simulink model "SPARCS_MIL"  (R2024a)
settings: Solver=VariableStepAuto  StartTime=0.0  StopTime=10.0  RelTol=1e-3
undefined symbols (not defined in the file or in its folder): attitude, epoch, IAU, juliandate, km, m, om0_x, om0_y, om0_z, s, satellite, simulator, WMM2020
libraries: simulink_extras x16, sharedtransform x14, SepehrMILLib x10, aerolibconvert2 x9, matrix_library x3, simulink x3, aerolibutil x3, vrlib x2, aerolibgravity2 x2, aerolibtransform2 x2
(part 1 of 2)
settings Model: Creator=dani  LastModifiedBy=dani

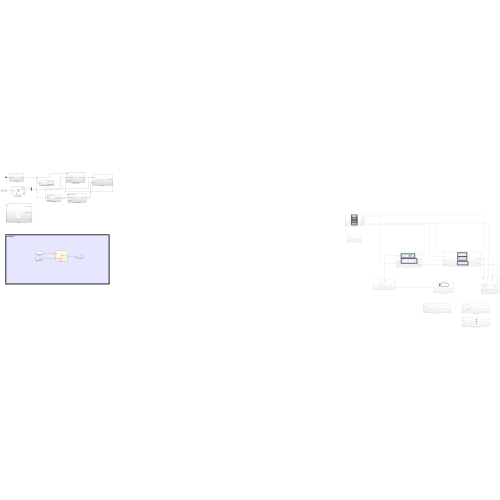
[thumbnail: Simulink's stored preview of the top-level diagram]
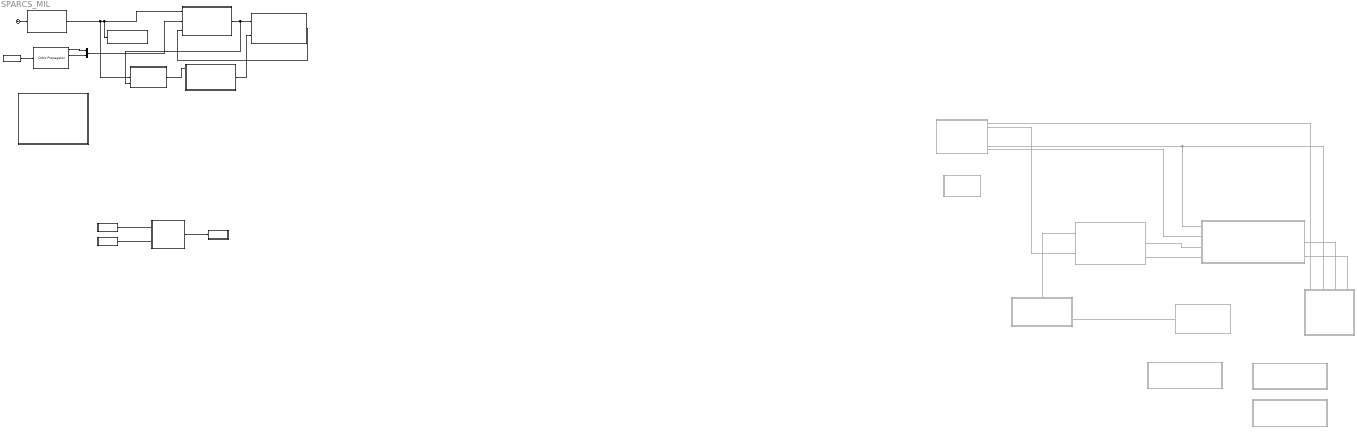
== system SPARCS_MIL ==
  note: Software
  Actuators : Subsystem  Commented=on
      settings: PortSchema="{\"entries\":[{\"content\":{\"sides\":[{\"content\":{},\"type\":\"ConnectorPlacement.EquallySpacedRectSide\",\"uuid\":\"57b5be20-0305-4655-b70d-f6d88ddf7cc3\"},{\"content\":{\"connectorIds\":[\"In1\",\"In2\"],\"side\":\"RIGHT\"},\"type\":\"ConnectorPlacement.EquallySpacedRectSide\",\"uuid\":\"30fbf78c-d5a5-42a2-90f1-8bab57c6ab77\"},{\"content\":{\"connectorIds\":[\"Out1\"],\"side\":\"TOP\"},\"type\":\"ConnectorPlacement.EquallySpacedRectSide\",\"uuid\":\"5a8d2e79-d609-4b0c-a176-c302cc1b65d1\"}]},\"type\":\"ConnectorPlacement.EquallySpacedConnector\",\"uuid\":\"3b08abd5-9373-451e-94da-caa467f9d6bd\"}],\"packageUris\":[\"http://schema.mathworks.com/mf0/Connector/R2020b\"],\"version\":\"1.0\"}"
  Attitude Control Algorithms : Subsystem  Commented=on
      settings: PortSchema="{\"entries\":[{\"content\":{\"sides\":[{\"content\":{\"connectorIds\":[\"Out1\"]},\"type\":\"ConnectorPlacement.EquallySpacedRectSide\",\"uuid\":\"41f8dcfc-afb1-4613-bda0-8bd0e5f6db23\"},{\"content\":{\"side\":\"RIGHT\"},\"type\":\"ConnectorPlacement.EquallySpacedRectSide\",\"uuid\":\"1cc831b3-3219-4888-a8b3-e3dddebb1701\"},{\"content\":{\"side\":\"TOP\"},\"type\":\"ConnectorPlacement.EquallySpacedRectSide\",\"uuid\":\"ddd3243b-04bb-419c-9fbc-88ec0dbe35ac\"}]},\"type\":\"ConnectorPlacement.EquallySpacedConnector\",\"uuid\":\"03796cc2-c9a7-47b9-b2cd-c3bab7a65dae\"}],\"packageUris\":[\"http://schema.mathworks.com/mf0/Connector/R2020b\"],\"version\":\"1.0\"}"
  Attitude Determination and Estimation Algorithms : Subsystem  Commented=on
      settings: PortSchema="{\"entries\":[{\"content\":{\"sides\":[{\"content\":{\"connectorIds\":[\"Out1\",\"Out2\",\"Out3\"]},\"type\":\"ConnectorPlacement.EquallySpacedRectSide\",\"uuid\":\"7b05d57f-a0cf-4401-a574-34b1755f21cb\"},{\"content\":{\"side\":\"RIGHT\"},\"type\":\"ConnectorPlacement.EquallySpacedRectSide\",\"uuid\":\"0f587f50-2c0a-47b1-bbff-e10884228d7f\"},{\"content\":{\"connectorIds\":[\"In1\",\"In2\",\"In3\",\"In4\"],\"side\":\"TOP\"},\"type\":\"ConnectorPlacement.EquallySpacedRectSide\",\"uuid\":\"7d75d2d9-c6c8-4539-b1b4-022bd2bc80cb\"},{\"content\":{\"side\":\"BOTTOM\"},\"type\":\"ConnectorPlacement.EquallySpacedRectSide\",\"uuid\":\"9e386f38-6887-4261-b78f-0a16f9b94efd\"}]},\"type\":\"ConnectorPlacement.EquallySpacedConnector\",\"uuid\":\"071a0923-cd7c-4dcb-a7b9-f4842b9df63f\"}],\"packageUris\":[\"http://schema.mathworks.com/mf0/Connector/R2020b\"],\"version\":\"1.0\"}"
  Attitude Dynamic : Subsystem
  Bus Creator : BusCreator  Inputs=2
  Calendar : Subsystem
  Clock : Clock
  Constant : Constant  Value=[0; 0; 0]
  Environment : Subsystem  Commented=on
  GNSS Receiver Model : Subsystem  Commented=on
  Gyroscope Model : Subsystem  Commented=on
  IGRF [ECEF] : Subsystem
  Kinematics and Dynamics : Subsystem  Commented=on
  Magnetometer Model : Subsystem  Commented=on
  Magnetorquers Model : Subsystem
  OBC : Stateflow chart  TreatAsAtomicUnit=on
  Orbit Propagator Numerical (high precision) : OrbitPropagator  propagator=Numerical (high precision)  accelIn=on  startDate=juliandate(epoch.Year, epoch.Month, epoch.Day, epoch.Hour, epoch.Minute, epoch.Second)  orbitType=Circular inclined  semiMajorAxis=6921000  inclination=55  raan=0  inertialPosition=[3649700.0 3308200.0 -4676600.0]  inertialVelocity=[-2750.8 6666.4 2573.4]  fixedPosition=[-4142689.0 -2676864.7 -4669861.6]  fixedVelocity=[1452.7 -6720.7 2568.1]  customR=3396200  customMu=4.305e13  customJ2=1.0826269e-03  customOmega=4.06125949e-3  outputTransform=on
  Planetary Ephemeris Calculator : Subsystem
  Reference Frames Transformations Manager : Subsystem
  Sensors : Subsystem
  Sensors1 : Subsystem  Commented=on
  Subsystem3 : Subsystem  Commented=on
  sensors sim : Subsystem
  telecommand receiver : Subsystem
  telemetry transponder : Subsystem
  wires:
  Environment/2(T_D(Body)) -> Kinematics and Dynamics/2(T_D(body))
  Kinematics and Dynamics/3(Omega(Body)[rad/s]) -> Sensors1/4(Omega(Body)[rad/s])
  Kinematics and Dynamics/2(q(ECI-Body)) -> Sensors1/3(q(ECI-Body))
  Environment/7(SunPos(ECI)) -> Attitude Determination and Estimation Algorithms/2(SunPos(ECI)), Sensors1/1(SunPos(ECI))
  Sensors1/2(B_meas(Body)[T]) -> Attitude Determination and Estimation Algorithms/3(B_Meas(Body))
  Sensors1/3(SunPos_Meas(Body)) -> Attitude Determination and Estimation Algorithms/4(SunPos_Meas(Body))
  Environment/8(Eclipse) -> Sensors1/2(Eclipse)
  Actuators/1(T_C(Body)) -> Kinematics and Dynamics/1(T_C(body))
  Environment/1(B(ECI)) -> Attitude Determination and Estimation Algorithms/1(B(ECI)[T])
  Attitude Control Algorithms/1(m) -> Actuators/2(m)
  Clock/1 -> Calendar/1(Since Epoch (sec))
  Calendar/1(Calendar) -> IGRF [ECEF]/2(Calendar), Planetary Ephemeris Calculator/1(Calendar), Reference Frames Transformations Manager/1(Calendar)
  Constant/1 -> Orbit Propagator Numerical (high precision)/1
  Orbit Propagator Numerical (high precision)/1 -> Bus Creator/1  "X"
  Orbit Propagator Numerical (high precision)/2 -> Bus Creator/2  "Y"
  Bus Creator/1 -> Reference Frames Transformations Manager/2(Ephemerides [ICRF])
  Reference Frames Transformations Manager/1(Transformers) -> IGRF [ECEF]/3(Transformers), Attitude Dynamic/1(Transformers)
  Attitude Dynamic/1(Satellite Attitude) -> Reference Frames Transformations Manager/3(Satellite Attitude)
  IGRF [ECEF]/1(Magnetic Field (T)) -> Magnetorquers Model/1(Magnetic Field [Body] (T))  "Magnetic Field (T)"
  Magnetorquers Model/1(Magnetorquers) -> Attitude Dynamic/2(Actuators)  "MTQs"
  sensors sim/1(Out1) -> OBC/1(sensors)
  telecommand receiver/1(telecommand) -> OBC/2(telecommand)
  OBC/1(telemetry) -> telemetry transponder/1(In1)

== system SPARCS_MIL/Actuators ==
  B(Body) : Inport
  m : Inport  Port=2
  A1 : Constant
  A2 : Constant
  Ax : Constant
  Cross Product : matrix_library/Cross Product
  Cross Product1 : matrix_library/Cross Product
  Cross Product2 : matrix_library/Cross Product
  Demux : Demux  Outputs=3
  Divide : Product  Inputs=*/
  Divide1 : Product  Inputs=*/
  Divide2 : Product  Inputs=*/
  Mux : Mux  Inputs=3
  N*A : Product
  N*A1 : Product
  N*A2 : Product
  N2 : Constant
  Nx : Constant
  Ny : Constant
  PWM : simulink/Discontinuities/PWM  DisableCoverage=on  Period=1  InitialDelay=0  DisallowZeroDutyCycle=off  RunAtFixedTimeIntervals=off  SampleTime=0.1
  PWM1 : simulink/Discontinuities/PWM  DisableCoverage=on  Period=1  InitialDelay=0  DisallowZeroDutyCycle=off  RunAtFixedTimeIntervals=off  SampleTime=0.1
  PWM2 : simulink/Discontinuities/PWM  DisableCoverage=on  Period=1  InitialDelay=0  DisallowZeroDutyCycle=off  RunAtFixedTimeIntervals=off  SampleTime=0.1
  Product : Product
  Product1 : Product
  Product2 : Product
  T_C(Body) : Outport
  wires:
  N*A2/1 -> Product2/2, Divide2/2
  Demux/1 -> Divide/1
  PWM2/1 -> Product2/1
  A1/1 -> N*A1/2
  Product1/1 -> Cross Product1/1  "m"
  Mux/1 -> T_C(Body)/1
  N2/1 -> N*A2/1
  Product2/1 -> Cross Product2/1  "m"
  Cross Product2/1 -> Mux/3
  PWM1/1 -> Product1/1
  A2/1 -> N*A2/2
  Divide1/1 -> PWM1/1  "i(Current)"
  Ax/1 -> N*A/2
  Divide/1 -> PWM/1  "i(Current)"
  Ny/1 -> N*A1/1
  Cross Product1/1 -> Mux/2
  N*A1/1 -> Product1/2, Divide1/2
  B(Body)/1 -> Cross Product2/2, Cross Product1/2, Cross Product/2  "B"
  m/1 -> Demux/1
  Demux/3 -> Divide2/1
  Demux/2 -> Divide1/1
  Nx/1 -> N*A/1
  N*A/1 -> Product/2, Divide/2
  Divide2/1 -> PWM2/1  "i(Current)"
  PWM/1 -> Product/1
  Product/1 -> Cross Product/1  "m"
  Cross Product/1 -> Mux/1

== system SPARCS_MIL/Attitude Control Algorithms ==
  m : Outport

== system SPARCS_MIL/Attitude Determination and Estimation Algorithms ==
  B(ECI)[T] : Inport
  SunPos(ECI) : Inport  Port=2
  B_Meas(Body) : Inport  Port=3
  SunPos_Meas(Body) : Inport  Port=4
  MATLAB Function : MATLAB Function  Commented=on  TreatAsAtomicUnit=on
  MATLAB Function1 : MATLAB Function  TreatAsAtomicUnit=on
  Cov_Matrix : Outport
  q_TRIAD(Body-ECI) : Outport  Port=2
  DCM_Mat(Body-ECI) : Outport  Port=3
  wires:
  SunPos(ECI)/1 -> MATLAB Function1/1(SunPos_ECI)
  B(ECI)[T]/1 -> MATLAB Function1/2(MagField_ECI)
  SunPos_Meas(Body)/1 -> MATLAB Function1/3(SunPos_Body)
  B_Meas(Body)/1 -> MATLAB Function1/4(MagField_Body)
  MATLAB Function1/1(quat_TRIAD) -> q_TRIAD(Body-ECI)/1
  MATLAB Function1/2(CovarianceMatrix) -> Cov_Matrix/1
  MATLAB Function1/3(RotationMatrix) -> DCM_Mat(Body-ECI)/1

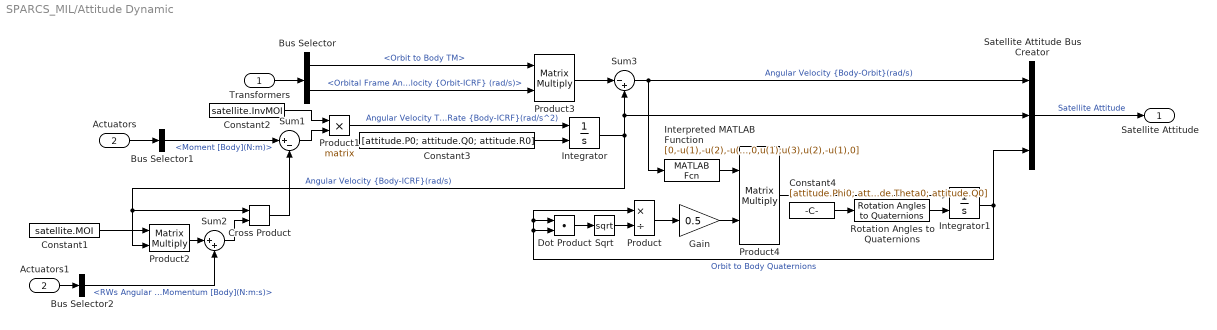
== system SPARCS_MIL/Attitude Dynamic ==
  Transformers : Inport
  Actuators : Inport  Port=2
  Actuators1 : InportShadow  Port=2
  Bus Selector : BusSelector  OutputSignals=Transfer Matrices.Orbit to Body TM,Orbital Elements.Orbital Frame Angular Velocity {Orbit-ICRF} (rad/s)
  Bus Selector1 : BusSelector  OutputSignals=Momenta [Body].Moment [Body](N:m)
  Bus Selector2 : BusSelector  OutputSignals=Momenta [Body].RWs Angular Momentum [Body](N:m:s)
  Constant1 : Constant  Value=satellite.MOI
  Constant2 : Constant  Value=satellite.InvMOI
  Constant3 : Constant  Value=[attitude.P0; attitude.Q0; attitude.R0]
  Constant4 : Constant  Value=[attitude.Phi0; attitude.Theta0; attitude.Q0]
  Cross Product : vrlib/Utilities/Cross Product
  Dot Product : DotProduct  OutDataTypeStr=Inherit: Inherit via internal rule
  Gain : Gain  Gain=0.5
  Integrator : Integrator  InitialConditionSource=external  ContinuousStateAttributes={'P','Q','R'}
  Integrator1 : Integrator  InitialConditionSource=external  ContinuousStateAttributes={'q0','q1','q2','q3'}
  Interpreted MATLAB Function : MATLABFcn  MATLABFcn=[0,-u(1),-u(2),-u(3);u(1),0,u(3),-u(2);u(2),-u(3),0,u(1);u(3),u(2),-u(1),0]  OutputDimensions=[4,4]  OutputSignalType=real  Output1D=off
  Product : Product  Inputs=*/
  Product{1..4} (4 alike) : Product  Multiplication=Matrix(*)
  Rotation Angles to Quaternions : sharedtransform/Rotation Angles to Quaternions  rotationOrder=XYZ  aMode=aMode
  Satellite Attitude Bus Creator : BusCreator  Inputs=3
  Sqrt : Sqrt  OutputSignalType=real
  Sum1 : Sum  Inputs=|+-
  Sum2 : Sum  Inputs=|++
  Sum3 : Sum  Inputs=|-+
  Satellite Attitude : Outport
  wires:
  Integrator/1 -> Cross Product/1, Product2/2, Satellite Attitude Bus Creator/2, Sum3/2  "Angular Velocity {Body-ICRF}(rad/s)"
  Bus Selector/2 -> Product3/2  "<Orbital Frame Angular Velocity {Orbit-ICRF} (rad/s)>"
  Constant2/1 -> Product1/1
  Interpreted MATLAB Function/1 -> Product4/1
  Bus Selector1/1 -> Sum1/1  "<Moment [Body](N:m)>"
  Constant1/1 -> Product2/1
  Dot Product/1 -> Sqrt/1
  Sqrt/1 -> Product/2
  Sum2/1 -> Cross Product/2
  Satellite Attitude Bus Creator/1 -> Satellite Attitude/1  "Satellite Attitude"
  Product3/1 -> Sum3/1
  Sum1/1 -> Product1/2
  Constant4/1 -> Rotation Angles to Quaternions/1
  Bus Selector2/1 -> Sum2/2  "<RWs Angular Momentum [Body](N:m:s)>"
  Cross Product/1 -> Sum1/2
  Transformers/1 -> Bus Selector/1
  Product1/1 -> Integrator/1  "Angular Velocity Time Rate {Body-ICRF}(rad/s^2)"
  Gain/1 -> Product4/2
  Actuators1/1 -> Bus Selector2/1
  Constant3/1 -> Integrator/2
  Product4/1 -> Integrator1/1
  Bus Selector/1 -> Product3/1  "<Orbit to Body TM>"
  Integrator1/1 -> Satellite Attitude Bus Creator/3, Dot Product/2, Product/1, Dot Product/1  "Orbit to Body Quaternions"
  Product2/1 -> Sum2/1
  Sum3/1 -> Satellite Attitude Bus Creator/1, Interpreted MATLAB Function/1  "Angular Velocity {Body-Orbit}(rad/s)"
  Actuators/1 -> Bus Selector1/1
  Rotation Angles to Quaternions/1 -> Integrator1/2
  Product/1 -> Gain/1

== system SPARCS_MIL/Calendar ==
  Since Epoch (sec) : Inport  OutDataTypeStr=double  Unit=s  PortDimensions=1
  Calendar Bus Creator : BusCreator  Inputs=4
  Constant6 : Constant  Value=epoch.DecimalYear
  JD : Subsystem
  MJD : Subsystem
  Calendar : Outport
  wires:
  Since Epoch (sec)/1 -> MJD/1(Since Epoch (sec)), JD/1(Since Epoch (sec)), Calendar Bus Creator/4  "Since Epoch (sec)"
  Constant6/1 -> Calendar Bus Creator/3  "Decimal Year (year)"
  JD/1(Julian Date (day)) -> Calendar Bus Creator/1  "Julian Date (day)"
  Calendar Bus Creator/1 -> Calendar/1  "Calendar"
  MJD/1(Modified Julian Date (day)) -> Calendar Bus Creator/2  "Modified Julian Date (day)"

== system SPARCS_MIL/Environment ==
  note: Eclipse(0 or 1)
  note: Orbit Propagator
  note: Earth Magnetic Field Model
  note: Perturbation
  note: Time
  note: Sun Vector
  lat : Inport
  lon : Inport  Port=2
  h : Inport  Port=3
  Clock : Clock
  Constant : Constant  Value=[3.2986e-5 3.2986e-5 3.2986e-5]
  Julian Date Conversion : aerolibconvert2/Julian Date Conversion  year=2020  month=January  day=1  hour=0  min=0  sec=0  modflag=off  deltaT=Sec  errorflag=Error
  Magnetic Field : Scope
  Orbit Propagator Numerical (high precision) : OrbitPropagator  propagator=Numerical (high precision)  inertialPosition=[3649700.0 3308200.0 -4676600.0]  inertialVelocity=[-2750.8 6666.4 2573.4]  fixedPosition=[-4142689.0 -2676864.7 -4669861.6]  fixedVelocity=[1452.7 -6720.7 2568.1]  customR=3396200  customMu=4.305e13  customJ2=1.0826269e-03  customOmega=4.06125949e-3  outputTransform=on
  Planetary Ephemeris : PlanetaryEphem  units=m,m/s  target=Sun
  Terminator : Terminator
  Terminator1 : Terminator
  Terminator2 : Terminator
  World Magnetic Model : aerolibgravity2/World Magnetic Model  model=WMM2020 (2020-2025)  customFile='WMM2020.COF'  units=Metric (MKS)  time_in=off  month=August  day=1  year=2024  action=Error  h_out=off  dec_out=on  inc_out=on  ti_out=off
  B(ECI) : Outport
  T_D(Body) : Outport  Port=2
  JD : Outport  Port=3
  X_Prop(ECI) : Outport  Port=4
  V_Prop(ECI) : Outport  Port=5
  q_ICRF2ff : Outport  Port=6
  SunPos(ECI) : Outport  Port=7
  Eclipse : Outport  Port=8
  wires:
  Planetary Ephemeris/2 -> Terminator2/1
  Orbit Propagator Numerical (high precision)/3 -> q_ICRF2ff/1
  Constant/1 -> T_D(Body)/1
  Planetary Ephemeris/1 -> SunPos(ECI)/1
  Orbit Propagator Numerical (high precision)/2 -> V_Prop(ECI)/1
  lat/1 -> World Magnetic Model/2
  Orbit Propagator Numerical (high precision)/1 -> X_Prop(ECI)/1
  Clock/1 -> Julian Date Conversion/1
  Julian Date Conversion/1 -> Planetary Ephemeris/1, JD/1
  World Magnetic Model/3 -> Terminator1/1
  World Magnetic Model/1 -> Magnetic Field/1, B(ECI)/1  "Manetic Field in  reference Frame"
  lon/1 -> World Magnetic Model/3
  h/1 -> World Magnetic Model/1  "Height"
  World Magnetic Model/2 -> Terminator/1

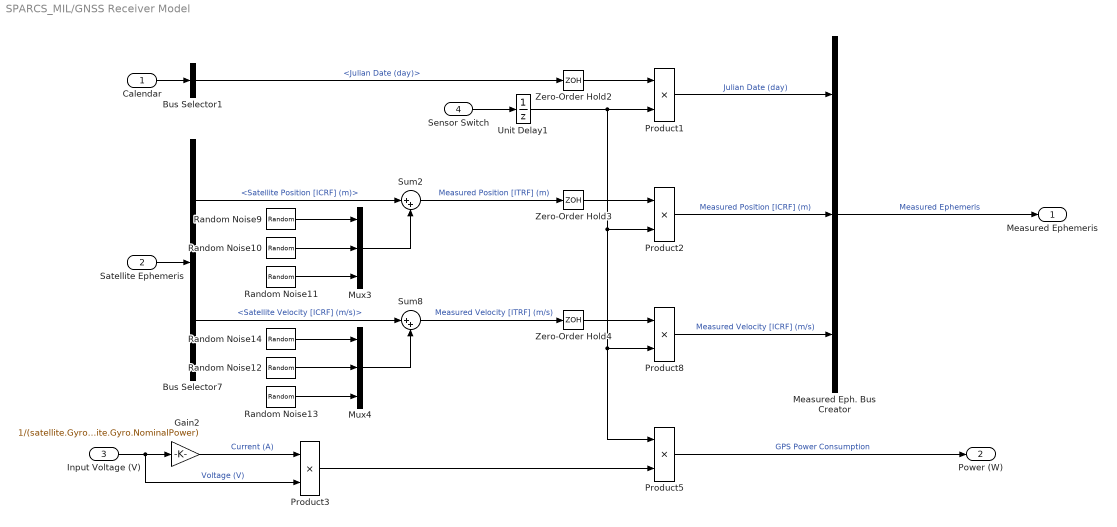
== system SPARCS_MIL/GNSS Receiver Model ==
  Calendar : Inport
  Satellite Ephemeris : Inport  Port=2
  Input Voltage (V) : Inport  Port=3
  Sensor Switch : Inport  Port=4
  Bus Selector1 : BusSelector  OutputSignals=Julian Date (day)
  Bus Selector7 : BusSelector  OutputSignals=Satellite Position [ICRF] (m),Satellite Velocity [ICRF] (m/s)
  Gain2 : Gain  Gain=1/(satellite.Gyro.NominalVoltage^2/satellite.Gyro.NominalPower)
  Measured Eph. Bus Creator : BusCreator  Inputs=3
  Mux3 : Mux  Inputs=3
  Mux4 : Mux  Inputs=3
  Product{1..3,5,8} (5 alike) : Product
  Random Noise10 : RandomNumber  Mean=satellite.GPS.Position.Bias  Variance=satellite.GPS.Position.NoiseSTDDEV^2  SampleTime=1/satellite.GPS.Frequency
  Random Noise11 : RandomNumber  Mean=satellite.GPS.Position.Bias  Variance=satellite.GPS.Position.NoiseSTDDEV^2  SampleTime=1/satellite.GPS.Frequency
  Random Noise12 : RandomNumber  Mean=satellite.GPS.Velocity.Bias  Variance=satellite.GPS.Position.NoiseSTDDEV^2  SampleTime=1/satellite.GPS.Frequency
  Random Noise13 : RandomNumber  Mean=satellite.GPS.Velocity.Bias  Variance=satellite.GPS.Position.NoiseSTDDEV^2  SampleTime=1/satellite.GPS.Frequency
  Random Noise14 : RandomNumber  Mean=satellite.GPS.Velocity.Bias  Variance=satellite.GPS.Position.NoiseSTDDEV^2  SampleTime=1/satellite.GPS.Frequency
  Random Noise9 : RandomNumber  Mean=satellite.GPS.Position.Bias  Variance=satellite.GPS.Position.NoiseSTDDEV^2  SampleTime=1/satellite.GPS.Frequency
  Sum2 : Sum  Inputs=|++
  Sum8 : Sum  Inputs=|++
  Unit Delay1 : UnitDelay  SampleTime=-1  HasFrameUpgradeWarning=on
  Zero-Order Hold2 : ZeroOrderHold  SampleTime=1/satellite.GPS.Frequency
  Zero-Order Hold3 : ZeroOrderHold  SampleTime=1/satellite.GPS.Frequency
  Zero-Order Hold4 : ZeroOrderHold  SampleTime=1/satellite.GPS.Frequency
  Measured Ephemeris : Outport
  Power (W) : Outport  Port=2
  wires:
  Product1/1 -> Measured Eph. Bus Creator/1  "Julian Date (day)"
  Random Noise12/1 -> Mux4/2
  Sum8/1 -> Zero-Order Hold4/1  "Measured Velocity [ITRF] (m/s)"
  Sensor Switch/1 -> Unit Delay1/1
  Zero-Order Hold3/1 -> Product2/1
  Product8/1 -> Measured Eph. Bus Creator/3  "Measured Velocity [ICRF] (m/s)"
  Measured Eph. Bus Creator/1 -> Measured Ephemeris/1  "Measured Ephemeris"
  Zero-Order Hold2/1 -> Product1/1
  Unit Delay1/1 -> Product1/2, Product2/2, Product8/2, Product5/1
  Product2/1 -> Measured Eph. Bus Creator/2  "Measured Position [ICRF] (m)"
  Product3/1 -> Product5/2
  Product5/1 -> Power (W)/1  "GPS Power Consumption"
  Random Noise9/1 -> Mux3/1
  Bus Selector7/2 -> Sum8/1  "<Satellite Velocity [ICRF] (m/s)>"
  Zero-Order Hold4/1 -> Product8/1
  Bus Selector7/1 -> Sum2/1  "<Satellite Position [ICRF] (m)>"
  Input Voltage (V)/1 -> Gain2/1, Product3/2  "Voltage (V)"
  Sum2/1 -> Zero-Order Hold3/1  "Measured Position [ITRF] (m)"
  Mux3/1 -> Sum2/2
  Random Noise10/1 -> Mux3/2
  Mux4/1 -> Sum8/2
  Random Noise11/1 -> Mux3/3
  Random Noise13/1 -> Mux4/3
  Bus Selector1/1 -> Zero-Order Hold2/1  "<Julian Date (day)>"
  Satellite Ephemeris/1 -> Bus Selector7/1
  Calendar/1 -> Bus Selector1/1
  Gain2/1 -> Product3/1  "Current (A)"
  Random Noise14/1 -> Mux4/1

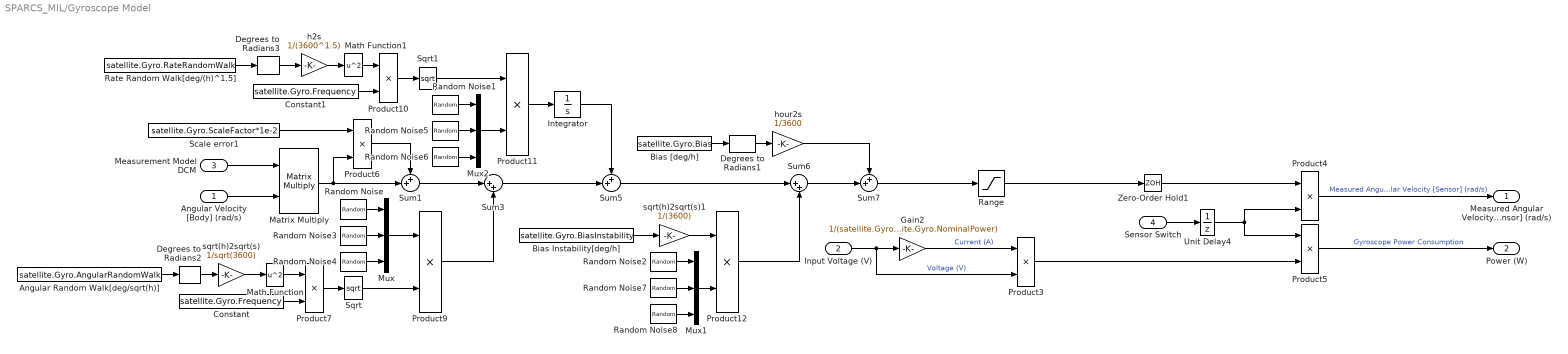
== system SPARCS_MIL/Gyroscope Model ==
  Angular Velocity [Body] (rad/s) : Inport
  Input Voltage (V) : Inport  Port=2
  Measurement Model DCM : Inport  Port=3
  Sensor Switch : Inport  Port=4
  Angular Random Walk[deg/sqrt(h)] : Constant  Value=satellite.Gyro.AngularRandomWalk
  Bias Instability[deg/h] : Constant  Value=satellite.Gyro.BiasInstability
  Bias [deg/h] : Constant  Value=satellite.Gyro.Bias
  Constant : Constant  Value=satellite.Gyro.Frequency
  Constant1 : Constant  Value=satellite.Gyro.Frequency
  Degrees to Radians1 : simulink_extras/Transformations/Degrees to Radians
  Degrees to Radians2 : simulink_extras/Transformations/Degrees to Radians
  Degrees to Radians3 : simulink_extras/Transformations/Degrees to Radians
  Gain2 : Gain  Gain=1/(satellite.Gyro.NominalVoltage^2/satellite.Gyro.NominalPower)
  Integrator : Integrator  InitialCondition=[0;0;0]
  Math Function : Math  Operator=square  SignedPower=on
  Math Function1 : Math  Operator=square  SignedPower=on
  Matrix Multiply : Product  Multiplication=Matrix(*)
  Mux : Mux  Inputs=3
  Mux1 : Mux  Inputs=3
  Mux2 : Mux  Inputs=3
  Product{3..7,9..12} (9 alike) : Product
  Random Noise{,1..8} (9 alike) : RandomNumber  SampleTime=1/satellite.Gyro.Frequency
  Range : Saturate  UpperLimit=satellite.Gyro.Range(2)  LowerLimit=satellite.Gyro.Range(1)
  Rate Random Walk[deg/(h)^1.5] : Constant  Value=satellite.Gyro.RateRandomWalk
  Scale error1 : Constant  Value=satellite.Gyro.ScaleFactor*1e-2
  Sqrt : Sqrt
  Sqrt1 : Sqrt
  Sum1 : Sum  Inputs=++|
  Sum3 : Sum  Inputs=|++
  Sum5 : Sum  Inputs=++|
  Sum6 : Sum  Inputs=|++
  Sum7 : Sum  Inputs=++|
  Unit Delay4 : UnitDelay  SampleTime=-1  HasFrameUpgradeWarning=on
  Zero-Order Hold1 : ZeroOrderHold  SampleTime=1/satellite.Gyro.Frequency
  h2s : Gain  Gain=1/(3600^1.5)
  hour2s : Gain  Gain=1/3600
  sqrt(h)2sqrt(s) : Gain  Gain=1/sqrt(3600)
  sqrt(h)2sqrt(s)1 : Gain  Gain=1/(3600)
  Measured Angular Velocity [Sensor] (rad/s) : Outport  PortDimensions=[3,1]
  Power (W) : Outport  Port=2
  wires:
  Sqrt/1 -> Product9/2
  Sum1/1 -> Sum3/1
  Sum6/1 -> Sum7/2
  hour2s/1 -> Sum7/1
  Matrix Multiply/1 -> Product6/2, Sum1/2
  Range/1 -> Zero-Order Hold1/1
  Random Noise3/1 -> Mux/2
  Mux/1 -> Product9/1
  Degrees to Radians3/1 -> h2s/1
  Product12/1 -> Sum6/2
  Product9/1 -> Sum3/2
  Product10/1 -> Sqrt1/1
  Random Noise5/1 -> Mux2/2
  Sum5/1 -> Sum6/1
  Integrator/1 -> Sum5/1
  Random Noise6/1 -> Mux2/3
  Math Function/1 -> Product7/1
  Random Noise7/1 -> Mux1/2
  sqrt(h)2sqrt(s)/1 -> Math Function/1
  Mux2/1 -> Product11/2
  Sum7/1 -> Range/1
  Angular Velocity [Body] (rad/s)/1 -> Matrix Multiply/2
  Product3/1 -> Product5/2
  Random Noise2/1 -> Mux1/1
  Constant/1 -> Product7/2
  Bias Instability[deg/h]/1 -> sqrt(h)2sqrt(s)1/1
  Random Noise4/1 -> Mux/3
  Angular Random Walk[deg/sqrt(h)]/1 -> Degrees to Radians2/1
  Gain2/1 -> Product3/1  "Current (A)"
  Random Noise/1 -> Mux/1
  Rate Random Walk[deg/(h)^1.5]/1 -> Degrees to Radians3/1
  Measurement Model DCM/1 -> Matrix Multiply/1
  Product6/1 -> Sum1/1
  Math Function1/1 -> Product10/1
  h2s/1 -> Math Function1/1
  Constant1/1 -> Product10/2
  Product7/1 -> Sqrt/1
  Scale error1/1 -> Product6/1
  Zero-Order Hold1/1 -> Product4/1
  Mux1/1 -> Product12/2
  Sqrt1/1 -> Product11/1
  Product11/1 -> Integrator/1
  Sum3/1 -> Sum5/2
  Sensor Switch/1 -> Unit Delay4/1
  sqrt(h)2sqrt(s)1/1 -> Product12/1
  Bias [deg/h]/1 -> Degrees to Radians1/1
  Degrees to Radians2/1 -> sqrt(h)2sqrt(s)/1
  Product4/1 -> Measured Angular Velocity [Sensor] (rad/s)/1  "Measured Angular Velocity [Sensor] (rad/s)"
  Degrees to Radians1/1 -> hour2s/1
  Random Noise1/1 -> Mux2/1
  Input Voltage (V)/1 -> Product3/2, Gain2/1  "Voltage (V)"
  Unit Delay4/1 -> Product5/1, Product4/2
  Product5/1 -> Power (W)/1  "Gyroscope Power Consumption"
  Random Noise8/1 -> Mux1/3

== system SPARCS_MIL/IGRF [ECEF] ==
  Satellite Position [ITRF] (m) : Inport
  Calendar : Inport  Port=2
  Transformers : Inport  Port=3
  Bus Selector : BusSelector  OutputSignals=Decimal Year (year)
  Bus Selector1 : BusSelector  OutputSignals=Transfer Matrices.ITRF to Body TM
  Convert to Teslla : Gain  Gain=10^-9  Multiplication=Matrix(K*u)
  Demux : Demux  Outputs=2
  Direction Cosine Matrix ECEF to NED : aerolibtransform2/Direction Cosine Matrix ECEF to NED
  Divide : Product  Inputs=**  Multiplication=Matrix(*)
  Divide1 : Product  Inputs=**  Multiplication=Matrix(*)
  ECEF Position to LLA : ECEF2LLA
  Magnetic Field Bus Creator : BusCreator  Inputs=2
  Mux : Mux  Inputs=2
  Reshape : Reshape  OutputDimensionality=Customize  OutputDimensions=[3,1]
  Transpose : Math  Operator=transpose
  World Magnetic Model : aerolibgravity2/World Magnetic Model  model=WMM2020 (2020-2025)  customFile='WMM2020.COF'  units=Metric (MKS)  time_in=on  month=January  day=1  year=2020  action=Error  h_out=off  dec_out=off  inc_out=off  ti_out=off
  Magnetic Field (T) : Outport  OutDataTypeStr=double  Unit=T
  wires:
  [Latitude_deg] -> World Magnetic Model/2  "Latitude (deg)"
  Transpose/1 -> Divide/1
  Demux/1 -> [Latitude_deg]
  [Altitude_m] -> World Magnetic Model/1  "Altitude (m)"
  Reshape/1 -> Magnetic Field Bus Creator/1, Divide1/2  "Magnetic Field (T) [ITRF]"
  Direction Cosine Matrix ECEF to NED/1 -> Transpose/1
  Magnetic Field Bus Creator/1 -> Magnetic Field (T)/1  "Magnetic Field (T)"
  Mux/1 -> Direction Cosine Matrix ECEF to NED/1
  Transformers/1 -> Bus Selector1/1
  [Latitude_deg] -> Mux/1  "Latitude (deg)"
  [Longitude_deg] -> Mux/2  "Longitude (deg)"
  ECEF Position to LLA/2 -> [Altitude_m]
  Demux/2 -> [Longitude_deg]
  Divide/1 -> Convert to Teslla/1
  Convert to Teslla/1 -> Reshape/1
  Calendar/1 -> Bus Selector/1
  ECEF Position to LLA/1 -> Demux/1
  Satellite Position [ITRF] (m)/1 -> ECEF Position to LLA/1  "Satellite Position [ITRF] (m)"
  [Longitude_deg] -> World Magnetic Model/3  "Longitude (deg)"
  Bus Selector/1 -> World Magnetic Model/4  "<Decimal Year (year)>"
  Divide1/1 -> Magnetic Field Bus Creator/2  "MagneticField (T)[Body]"
  World Magnetic Model/1 -> Divide/2
  Bus Selector1/1 -> Divide1/1  "<ITRF to Body TM>"

== system SPARCS_MIL/Kinematics and Dynamics ==
  note: Custom
  note: Force applied to the spacecraft center of mass in the body frame
  note: Prebuilt
  note: Moment applied to the spacecraft center of mass in the body frame
  T_C(body) : Inport
  T_D(body) : Inport  Port=2
  Demux : Demux  Outputs=3
  Dynamics : Subsystem
  ECI Position to LLA : aerolibtransform2/ECI Position to LLA  red=IAU-2000/2006  year=2013  month=January  day=1  hour=0  min=0  sec=0  deltaT=Day  errorflag=Error  extraparamflag=off  eunits=Metric (MKS)  earthmodel=WGS84  flat=1/298.257223563  eqradius=6378137
      settings: AttributesFormatString=%<red>
  F_body : Constant  Value=[0 0 0]
  Moment of Inertia Matrix : Constant  Value=[0.0013 0.0016 0.0014]
  Spacecraft Dynamics : SpacecraftDynamics  accelIn=on  mass=2.8  stateFormatNum=Fixed-frame state vector  semiMajorAxis=6921000  eccentricity=0  inclination=55  raan=0  argPeriapsis=0  trueAnomaly=0
  Sum : Sum  Inputs=|++
  Terminator{,1..6} (7 alike) : Terminator
  kinematics : Subsystem
  om_body : Scope
  X(ECI)[m] : Outport
  q(ECI-Body) : Outport  Port=2
  Omega(Body)[rad/s] : Outport  Port=3
  wires:
  Demux/3 -> Terminator3/1  "h"
  Demux/1 -> Terminator1/1  "lat"
  Spacecraft Dynamics/5 -> Terminator4/1, ECI Position to LLA/2  "UTC"
  Spacecraft Dynamics/2 -> Terminator6/1  "V(ECI)[m/s]"
  Demux/2 -> Terminator2/1  "lon"
  ECI Position to LLA/1 -> Demux/1
  Spacecraft Dynamics/4 -> Terminator5/1  "Omega(ECI-Body)"
  Moment of Inertia Matrix/1 -> Dynamics/2(I)
  Spacecraft Dynamics/3 -> q(ECI-Body)/1
  T_D(body)/1 -> Sum/2  "T_D(body)"
  T_C(body)/1 -> Sum/1  "T_C(body)"
  Sum/1 -> Dynamics/1(T_body), Spacecraft Dynamics/2  "T(body)"
  F_body/1 -> Spacecraft Dynamics/1
  kinematics/1(Out1) -> Terminator/1
  Spacecraft Dynamics/1 -> ECI Position to LLA/1, X(ECI)[m]/1
  Dynamics/1(om) -> Omega(Body)[rad/s]/1, om_body/1, kinematics/1(om)

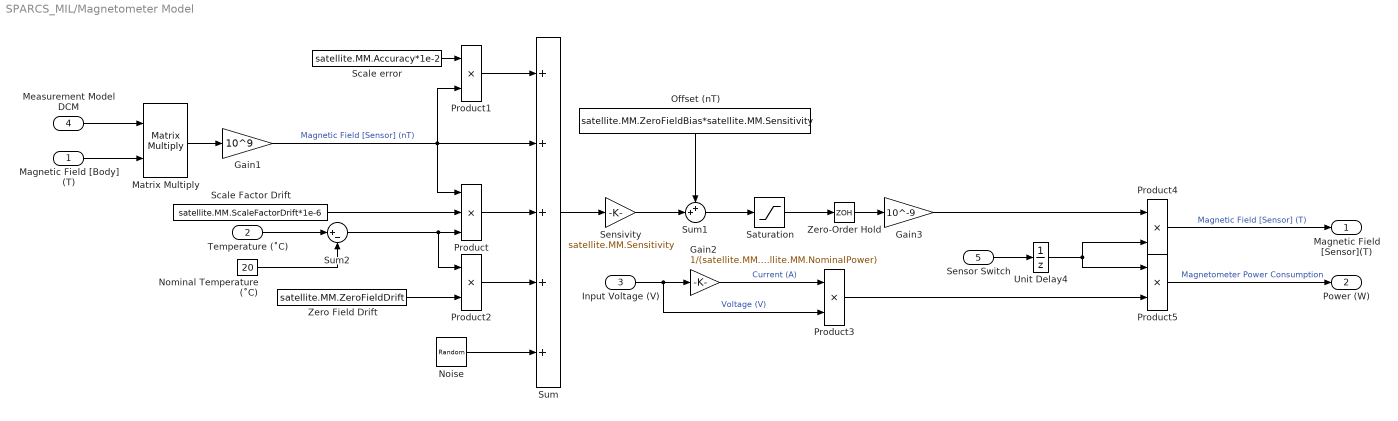
== system SPARCS_MIL/Magnetometer Model ==
  Magnetic Field [Body] (T) : Inport
  Temperature (˚C) : Inport  Port=2
  Input Voltage (V) : Inport  Port=3
  Measurement Model DCM : Inport  Port=4
  Sensor Switch : Inport  Port=5
  Gain1 : Gain  Gain=10^9
  Gain2 : Gain  Gain=1/(satellite.MM.NominalVoltage^2/satellite.MM.NominalPower)
  Gain3 : Gain  Gain=10^-9
  Matrix Multiply : Product  Multiplication=Matrix(*)
  Noise : RandomNumber  Variance=satellite.MM.NoiseVariance  SampleTime=1/satellite.MM.Frequency
  Nominal Temperature (˚C) : Constant  Value=20
  Offset (nT) : Constant  Value=satellite.MM.ZeroFieldBias*satellite.MM.Sensitivity
  Product : Product  Inputs=3
  Product{1..5} (5 alike) : Product
  Saturation : Saturate  UpperLimit=satellite.MM.Range(2)  LowerLimit=satellite.MM.Range(1)
  Scale Factor Drift : Constant  Value=satellite.MM.ScaleFactorDrift*1e-6
  Scale error : Constant  Value=satellite.MM.Accuracy*1e-2
  Sensivity : Gain  Gain=satellite.MM.Sensitivity
  Sum : Sum  Inputs=+++++
  Sum1 : Sum  Inputs=++|
  Sum2 : Sum  Inputs=|+-
  Unit Delay4 : UnitDelay  SampleTime=-1  HasFrameUpgradeWarning=on
  Zero Field Drift : Constant  Value=satellite.MM.ZeroFieldDrift
  Zero-Order Hold : ZeroOrderHold  SampleTime=1/satellite.MM.Frequency
  Magnetic Field [Sensor](T) : Outport  PortDimensions=[3,1]
  Power (W) : Outport  Port=2
  wires:
  Product3/1 -> Product5/2
  Scale error/1 -> Product1/1
  Sum2/1 -> Product/3, Product2/1
  Saturation/1 -> Zero-Order Hold/1
  Product2/1 -> Sum/4
  Zero-Order Hold/1 -> Gain3/1
  Nominal Temperature (˚C)/1 -> Sum2/2
  Gain2/1 -> Product3/1  "Current (A)"
  Offset (nT)/1 -> Sum1/1
  Measurement Model DCM/1 -> Matrix Multiply/1
  Temperature (˚C)/1 -> Sum2/1
  Product/1 -> Sum/3
  Product1/1 -> Sum/1
  Sensor Switch/1 -> Unit Delay4/1
  Input Voltage (V)/1 -> Gain2/1, Product3/2  "Voltage (V)"
  Sum/1 -> Sensivity/1
  Zero Field Drift/1 -> Product2/2
  Product4/1 -> Magnetic Field [Sensor](T)/1  "Magnetic Field [Sensor] (T)"
  Scale Factor Drift/1 -> Product/2
  Noise/1 -> Sum/5
  Gain1/1 -> Product1/2, Product/1, Sum/2  "Magnetic Field [Sensor] (nT)"
  Sum1/1 -> Saturation/1
  Sensivity/1 -> Sum1/2
  Magnetic Field [Body] (T)/1 -> Matrix Multiply/2
  Gain3/1 -> Product4/1
  Unit Delay4/1 -> Product4/2, Product5/1
  Matrix Multiply/1 -> Gain1/1
  Product5/1 -> Power (W)/1  "Magnetometer Power Consumption"

== system SPARCS_MIL/Magnetorquers Model ==
  Magnetic Field [Body] (T) : Inport
  MTQ CMD (A.m^2) : Inport  Port=2  PortDimensions=[3,1]
  MTQ Switches : Inport  Port=3  PortDimensions=[3,1]
  Abs : Abs  SaturateOnIntegerOverflow=off
  Abs1 : Abs  SaturateOnIntegerOverflow=off
  Constant : Constant
  Constant1 : Constant
  Cross Product : vrlib/Utilities/Cross Product
  Dot Product : DotProduct  OutDataTypeStr=Inherit: Inherit via internal rule
  Gain : Gain  Gain=0.5
  Gain1 : Gain  Gain=-1
  Gain2 : Gain  Gain=0.5
  Magnetorquers Bus Creator : BusCreator  Inputs=3
  Nominal Dipole : Constant  Value=satellite.MTQ.DPMoment
  Nominal Dipole1 : Constant  Value=satellite.MTQ.DPMoment
  Power : Constant  Value=satellite.MTQ.Power
  Product : Product  Inputs=3
  Product1 : Product  Inputs=*/
  Product2 : Product
  Product3 : Product
  Sign : Signum
  Sign1 : Signum
  Sign2 : Signum
  Sum : Sum  Inputs=|+-
  Sum1 : Sum  Inputs=|++
  Sum2 : Sum  Inputs=++|
  Sum3 : Sum  Inputs=|++
  Magnetorquers : Outport
  wires:
  Product3/1 -> Product1/1, Sign1/1, Product2/1, Abs/1
  Product2/1 -> Sum3/1
  Product1/1 -> Abs1/1
  Gain/1 -> Product/2
  Abs1/1 -> Dot Product/1
  Product/1 -> Sum3/2
  Sum1/1 -> Gain/1
  Nominal Dipole/1 -> Product/3, Sum/2
  Sign/1 -> Sum1/1
  Dot Product/1 -> Magnetorquers Bus Creator/3  "Power (W)"
  Magnetic Field [Body] (T)/1 -> Cross Product/2
  Abs/1 -> Sum/1
  MTQ Switches/1 -> Product3/2
  Gain2/1 -> Product2/2
  Power/1 -> Dot Product/2
  Sum3/1 -> Magnetorquers Bus Creator/1, Cross Product/1  "Dipoles (A.m^2)"
  Nominal Dipole1/1 -> Product1/2
  Sum2/1 -> Gain2/1
  Sign2/1 -> Sum2/2
  Constant1/1 -> Sum2/1
  Sum/1 -> Sign/1, Gain1/1
  MTQ CMD (A.m^2)/1 -> Product3/1
  Magnetorquers Bus Creator/1 -> Magnetorquers/1  "Magnetorquers"
  Constant/1 -> Sum1/2
  Cross Product/1 -> Magnetorquers Bus Creator/2  "CoilsTorque [Body] (N.m)"
  Sign1/1 -> Product/1
  Gain1/1 -> Sign2/1

== system SPARCS_MIL/OBC/boot. ==
  Action Port : ActionPort
      settings: CopyFcn=Stateflow.SLINSF.SimulinkMan.removeBlockPreDeleteFcn  PreDeleteFcn=Stateflow.SLINSF.SimulinkMan.unsafePredeleteFcn

== system SPARCS_MIL/OBC/running.nominal.detum.detumb_soft ==
  telecommand : Inport
  Action Port : ActionPort
      settings: CopyFcn=Stateflow.SLINSF.SimulinkMan.removeBlockPreDeleteFcn  PreDeleteFcn=Stateflow.SLINSF.SimulinkMan.unsafePredeleteFcn
  ADCS : Subsystem
  Telecommand digest : Subsystem
  power : Subsystem
  wires:
  Telecommand digest/1(Out1) -> ADCS/1(In1)
  Telecommand digest/2(Out2) -> power/1(In1)
  telecommand/1 -> Telecommand digest/1(telecommand)

== system SPARCS_MIL/Planetary Ephemeris Calculator ==
  Calendar : Inport
  Bus Selector : BusSelector  OutputSignals=Julian Date (day)
  Length Conversion : aerolibconvert2/Length Conversion  IU=km  OU=m
  Length Conversion1 : aerolibconvert2/Length Conversion  IU=km  OU=m
  Moon Ephemeris Bus Creator : BusCreator  Inputs=2
  Moon Ephemeris Calculator : PlanetaryEphem
  Sun Ephemeris Bus Creator : BusCreator  Inputs=2
  Sun Ephemeris Calculator : PlanetaryEphem  target=Sun
  Velocity Conversion : aerolibconvert2/Velocity Conversion  IU=km/s  OU=m/s
  Velocity Conversion1 : aerolibconvert2/Velocity Conversion  IU=km/s  OU=m/s
  Moon Ephemeris [ICRF] : Outport
  Sun Ephemeris [ICRF] : Outport  Port=2
  wires:
  Moon Ephemeris Bus Creator/1 -> Moon Ephemeris [ICRF]/1  "Moon Ephemeris [ICRF]"
  Velocity Conversion/1 -> Moon Ephemeris Bus Creator/2  "Moon Velocity [ICRF] (m/s)"
  Bus Selector/1 -> Moon Ephemeris Calculator/1, Sun Ephemeris Calculator/1  "<Julian Date (day)>"
  Moon Ephemeris Calculator/2 -> Velocity Conversion/1
  Calendar/1 -> Bus Selector/1
  Sun Ephemeris Calculator/1 -> Length Conversion1/1
  Sun Ephemeris Calculator/2 -> Velocity Conversion1/1
  Velocity Conversion1/1 -> Sun Ephemeris Bus Creator/2  "Sun Velocity [ICRF] (m/s)"
  Length Conversion/1 -> Moon Ephemeris Bus Creator/1  "Moon Position [ICRF] (m)"
  Sun Ephemeris Bus Creator/1 -> Sun Ephemeris [ICRF]/1  "Sun Ephemeris [ICRF]"
  Length Conversion1/1 -> Sun Ephemeris Bus Creator/1  "Sun Position [ICRF] (m)"
  Moon Ephemeris Calculator/1 -> Length Conversion/1

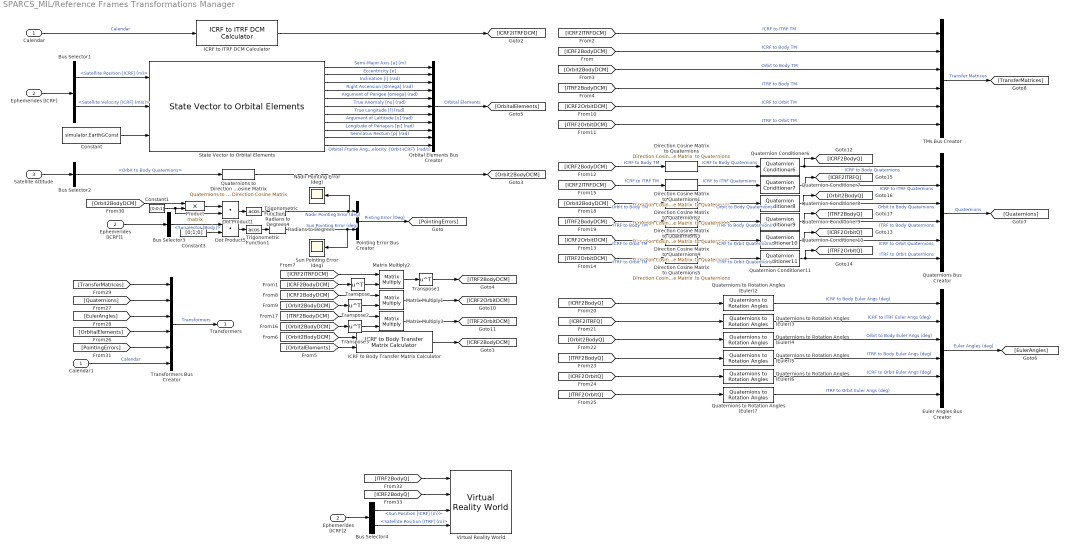
== system SPARCS_MIL/Reference Frames Transformations Manager ==
  Calendar : Inport
  Ephemerides [ICRF] : Inport  Port=2
  Satellite Attitude : Inport  Port=3
  Bus Selector1 : BusSelector  OutputSignals=Satellite Ephemeris [ICRF].Satellite Position [ICRF] (m),Satellite Ephemeris [ICRF].Satellite Velocity [ICRF] (m/s)
  Bus Selector2 : BusSelector  OutputSignals=Orbit to Body Quaternions
  Bus Selector3 : BusSelector  OutputSignals=Satellite Ephemeris [ICRF].Sun Vector [Body]
  Bus Selector4 : BusSelector  OutputSignals=Sun Ephemeris [ICRF].Sun Position [ICRF] (m),Satellite Ephemeris [ICRF].Satellite Position [ITRF] (m)
  Calendar1 : InportShadow
  Constant : Constant  Value=simulator.EarthGConst
  Constant1 : Constant  Value=[0;0;1]
  Constant3 : Constant  Value=[0;1;0]
  Direction Cosine Matrix to Quaternions{,1..5} (6 alike) : sharedtransform/Direction Cosine Matrix  to Quaternions  aMode=0  action=None  tolerance=eps(2)
  Dot Product1 : DotProduct  OutDataTypeStr=Inherit: Inherit via internal rule
  Dot Product5 : DotProduct  OutDataTypeStr=Inherit: Inherit via internal rule
  Ephemerides [ICRF]1 : InportShadow  Port=2
  Ephemerides [ICRF]2 : InportShadow  Port=2
  Euler Angles Bus Creator : BusCreator  Inputs=6
  ICRF to Body Transfer Matrix Calculator : SepehrMILLib/Reference Frames Transformations Manager/ICRF to Body Transfer Matrix Calculator  SystemSampleTime=-1  VariantActivationTime=update diagram  AllowFlexibleInterface=on  Latency=0  AutoFrameSizeCalculation=off
  ICRF to ITRF DCM Calculator : SepehrMILLib/Reference Frames Transformations Manager/ICRF to ITRF DCM Calculator  SystemSampleTime=-1  VariantActivationTime=update diagram  AllowFlexibleInterface=on  Latency=0  AutoFrameSizeCalculation=off
  Matrix Multiply1 : Product  Multiplication=Matrix(*)
  Matrix Multiply2 : Product  Multiplication=Matrix(*)
  Matrix Multiply3 : Product  Multiplication=Matrix(*)
  Nadir Pointing Error (deg) : Scope
  Orbital Elements Bus Creator : BusCreator  Inputs=11
  Pointing Error Bus Creator : BusCreator  Inputs=2
  Product : Product  Multiplication=Matrix(*)
  Quaternion Conditioner10 : SepehrMILLib/Reference Frames Transformations Manager/Quaternion Conditioner10  SystemSampleTime=-1  VariantActivationTime=update diagram  AllowFlexibleInterface=on  Latency=0  AutoFrameSizeCalculation=off
  Quaternion Conditioner11 : SepehrMILLib/Reference Frames Transformations Manager/Quaternion Conditioner11  SystemSampleTime=-1  VariantActivationTime=update diagram  AllowFlexibleInterface=on  Latency=0  AutoFrameSizeCalculation=off
  Quaternion Conditioner6 : SepehrMILLib/Reference Frames Transformations Manager/Quaternion Conditioner6  SystemSampleTime=-1  VariantActivationTime=update diagram  AllowFlexibleInterface=on  Latency=0  AutoFrameSizeCalculation=off
  Quaternion Conditioner7 : SepehrMILLib/Reference Frames Transformations Manager/Quaternion Conditioner7  SystemSampleTime=-1  VariantActivationTime=update diagram  AllowFlexibleInterface=on  Latency=0  AutoFrameSizeCalculation=off
  Quaternion Conditioner8 : SepehrMILLib/Reference Frames Transformations Manager/Quaternion Conditioner8  SystemSampleTime=-1  VariantActivationTime=update diagram  AllowFlexibleInterface=on  Latency=0  AutoFrameSizeCalculation=off
  Quaternion Conditioner9 : SepehrMILLib/Reference Frames Transformations Manager/Quaternion Conditioner9  SystemSampleTime=-1  VariantActivationTime=update diagram  AllowFlexibleInterface=on  Latency=0  AutoFrameSizeCalculation=off
  Quaternions Bus Creator : BusCreator  Inputs=6
  Quaternions to Direction Cosine Matrix : sharedtransform/Quaternions to  Direction Cosine Matrix  aMode=aMode
  Quaternions to Rotation Angles (Euler){2..7} (6 alike) : sharedtransform/Quaternions to Rotation Angles  rotationOrder=XYZ  aMode=aMode
  Radians to Degrees : simulink_extras/Transformations/Radians to Degrees
  Radians to Degrees4 : simulink_extras/Transformations/Radians to Degrees
  State Vector to Orbital Elements : SepehrMILLib/Reference Frames Transformations Manager/State Vector to Orbital Elements  SystemSampleTime=-1  VariantActivationTime=update diagram  AllowFlexibleInterface=on  Latency=0  AutoFrameSizeCalculation=off
  Sun Pointing Error (deg) : Scope
  TMs Bus Creator : BusCreator  Inputs=6
  Transformers Bus Creator : BusCreator  Inputs=6
  Transpose{,1..3} (4 alike) : Math  Operator=transpose
  Trigonometric Function : Trigonometry  Operator=acos
  Trigonometric Function1 : Trigonometry  Operator=acos  OutputSignalType=real
  Virtual Reality World : SepehrMILLib/Reference Frames Transformations Manager/Virtual Reality World  SystemSampleTime=-1  VariantControl=visSL3D  VariantActivationTime=update diagram  AllowFlexibleInterface=on  Latency=0  AutoFrameSizeCalculation=off
  Transformers : Outport
  wires:
  State Vector to Orbital Elements/7 -> Orbital Elements Bus Creator/7  "True Longitude [l] (rad)"
  Quaternion Conditioner8/1 -> Quaternions Bus Creator/3, [Orbit2BodyQ]  "Orbit to Body Quaternions"
  [Orbit2BodyQ] -> Quaternions to Rotation Angles (Euler)4/1
  [ITRF2OrbitQ] -> Quaternions to Rotation Angles (Euler)7/1
  [ITRF2OrbitDCM] -> Direction Cosine Matrix to Quaternions5/1  "ITRF to Orbit TM"
  Bus Selector1/2 -> State Vector to Orbital Elements/2  "<Satellite Velocity [ICRF] (m/s)>"
  [ICRF2ITRFQ] -> Quaternions to Rotation Angles (Euler)3/1
  [Orbit2BodyDCM] -> Transpose3/1
  [ICRF2OrbitQ] -> Quaternions to Rotation Angles (Euler)6/1
  [ICRF2BodyDCM] -> Matrix Multiply1/1
  [EulerAngles] -> Transformers Bus Creator/3
  State Vector to Orbital Elements/6 -> Orbital Elements Bus Creator/6  "True Anomaly [nu] (rad)"
  State Vector to Orbital Elements/5 -> Orbital Elements Bus Creator/5  "Argument of Perigee [omega] (rad)"
  Bus Selector4/1 -> Virtual Reality World/3  "<Sun Position [ICRF] (m)>"
  Transformers Bus Creator/1 -> Transformers/1  "Transformers"
  State Vector to Orbital Elements/4 -> Orbital Elements Bus Creator/4  "Right Ascension [Omega] (rad)"
  State Vector to Orbital Elements/10 -> Orbital Elements Bus Creator/10  "Semilatus Rectum [p] (rad)"
  State Vector to Orbital Elements/9 -> Orbital Elements Bus Creator/9  "Longitude of Periapsis [pi] (rad)"
  Quaternion Conditioner10/1 -> Quaternions Bus Creator/5, [ICRF2OrbitQ]  "ICRF to Orbit Quaternions"
  State Vector to Orbital Elements/8 -> Orbital Elements Bus Creator/8  "Argument of Lattitude [u] (rad)"
  Quaternions to Direction Cosine Matrix/1 -> [Orbit2BodyDCM]
  State Vector to Orbital Elements/1 -> Orbital Elements Bus Creator/1  "Semi-Major Axis [a] (m)"
  [OrbitalElements] -> ICRF to Body Transfer Matrix Calculator/2
  Ephemerides [ICRF]1/1 -> Bus Selector3/1
  Dot Product5/1 -> Trigonometric Function1/1
  [ICRF2BodyDCM] -> Transpose/1
  Matrix Multiply2/1 -> Transpose1/1
  [ITRF2BodyQ] -> Virtual Reality World/1
  Bus Selector1/1 -> State Vector to Orbital Elements/1  "<Satellite Position [ICRF] (m)>"
  ICRF to Body Transfer Matrix Calculator/1 -> [ICRF2BodyDCM]
  Transpose2/1 -> Matrix Multiply1/2
  ICRF to ITRF DCM Calculator/1 -> [ICRF2ITRFDCM]
  Orbital Elements Bus Creator/1 -> [OrbitalElements]  "Orbital Elements"
  Transpose1/1 -> [ITRF2BodyDCM]
  Trigonometric Function/1 -> Radians to Degrees4/1
  Matrix Multiply3/1 -> [ITRF2OrbitDCM]
  Constant3/1 -> Dot Product5/2
  [OrbitalElements] -> Transformers Bus Creator/4
  [ITRF2BodyDCM] -> Matrix Multiply3/1
  Transpose3/1 -> Matrix Multiply3/2
  Radians to Degrees4/1 -> Pointing Error Bus Creator/1, Nadir Pointing Error (deg)/1  "Nadir Pointing Error (deg)"
  Radians to Degrees/1 -> Sun Pointing Error (deg)/1, Pointing Error Bus Creator/2  "Sun Pointing Error (deg)"
  Calendar/1 -> ICRF to ITRF DCM Calculator/1  "Calendar"
  Bus Selector4/2 -> Virtual Reality World/4  "<Satellite Position [ITRF] (m)>"
  Pointing Error Bus Creator/1 -> [PointingErrors]  "Pinting Error (Deg)"
  [ICRF2BodyQ] -> Virtual Reality World/2
  State Vector to Orbital Elements/11 -> Orbital Elements Bus Creator/11  "Orbital Frame Angular Velocity {Orbit-ICRF} (rad/s)"
  Constant/1 -> State Vector to Orbital Elements/3
  [Orbit2BodyDCM] -> Direction Cosine Matrix to Quaternions2/1  "Orbit to Body TM"
  [ICRF2ITRFDCM] -> TMs Bus Creator/1  "ICRF to ITRF TM"
  [ICRF2BodyDCM] -> TMs Bus Creator/2  "ICRF to Body TM"
  [PointingErrors] -> Transformers Bus Creator/5
  Transpose/1 -> Matrix Multiply2/2
  [Orbit2BodyDCM] -> Product/1
  Direction Cosine Matrix to Quaternions/1 -> Quaternion Conditioner6/1  "ICRF to Body Quaternions"
  [ICRF2OrbitDCM] -> TMs Bus Creator/5  "ICRF to Orbit TM"
  Quaternion Conditioner11/1 -> Quaternions Bus Creator/6, [ITRF2OrbitQ]  "ITRF to Orbit Quaternions"
  Direction Cosine Matrix to Quaternions3/1 -> Quaternion Conditioner9/1  "ITRF to Body Quaternions"
  [ICRF2BodyQ] -> Quaternions to Rotation Angles (Euler)2/1
  Constant1/1 -> Product/2, Dot Product1/2
  [ITRF2BodyDCM] -> TMs Bus Creator/4  "ITRF to Body TM"
  Quaternions to Rotation Angles (Euler)7/1 -> Euler Angles Bus Creator/6  "ITRF to Orbit Euler Angs (deg)"
  [Quaternions] -> Transformers Bus Creator/2
  [ITRF2OrbitDCM] -> TMs Bus Creator/6  "ITRF to Orbit TM"
  [ICRF2ITRFDCM] -> Matrix Multiply2/1
  Satellite Attitude/1 -> Bus Selector2/1
  Calendar1/1 -> Transformers Bus Creator/6  "Calendar"
  State Vector to Orbital Elements/2 -> Orbital Elements Bus Creator/2  "Eccentricity [e]"
  Quaternion Conditioner7/1 -> Quaternions Bus Creator/2, [ICRF2ITRFQ]  "ICRF to ITRF Quaternions"
  Ephemerides [ICRF]/1 -> Bus Selector1/1
  Quaternions Bus Creator/1 -> [Quaternions]  "Quaternions"
  [ICRF2ITRFDCM] -> Direction Cosine Matrix to Quaternions1/1  "ICRF to ITRF TM"
  Matrix Multiply1/1 -> [ICRF2OrbitDCM]
  Ephemerides [ICRF]2/1 -> Bus Selector4/1
  Direction Cosine Matrix to Quaternions5/1 -> Quaternion Conditioner11/1  "ITRF to Orbit Quaternions"
  Direction Cosine Matrix to Quaternions4/1 -> Quaternion Conditioner10/1  "ICRF to Orbit Quaternions"
  TMs Bus Creator/1 -> [TransferMatrices]  "Transfer Matrices"
  [ITRF2BodyDCM] -> Direction Cosine Matrix to Quaternions3/1  "ITRF to Body TM"
  Bus Selector3/1 -> Dot Product5/1  "<Sun Vector [Body]>"
  Product/1 -> Dot Product1/1
  Bus Selector2/1 -> Quaternions to Direction Cosine Matrix/1  "<Orbit to Body Quaternions>"
  [Orbit2BodyDCM] -> Transpose2/1
  Quaternion Conditioner9/1 -> Quaternions Bus Creator/4, [ITRF2BodyQ]  "ITRF to Body Quaternions"
  Direction Cosine Matrix to Quaternions2/1 -> Quaternion Conditioner8/1  "Orbit to Body Quaternions"
  Quaternion Conditioner6/1 -> Quaternions Bus Creator/1, [ICRF2BodyQ]  "ICRF to Body Quaternions"
  Quaternions to Rotation Angles (Euler)5/1 -> Euler Angles Bus Creator/4  "ITRF to Body Euler Angs (deg)"
  Dot Product1/1 -> Trigonometric Function/1
  Direction Cosine Matrix to Quaternions1/1 -> Quaternion Conditioner7/1  "ICRF to ITRF Quaternions"
  Quaternions to Rotation Angles (Euler)2/1 -> Euler Angles Bus Creator/1  "ICRF to Body Euler Angs (deg)"
  Quaternions to Rotation Angles (Euler)3/1 -> Euler Angles Bus Creator/2  "ICRF to ITRF Euler Angs (deg)"
  Euler Angles Bus Creator/1 -> [EulerAngles]  "Euler Angles (deg)"
  State Vector to Orbital Elements/3 -> Orbital Elements Bus Creator/3  "Inclination [i] (rad)"
  [TransferMatrices] -> Transformers Bus Creator/1
  [ICRF2OrbitDCM] -> Direction Cosine Matrix to Quaternions4/1  "ICRF to Orbit TM"
  Quaternions to Rotation Angles (Euler)6/1 -> Euler Angles Bus Creator/5  "ICRF to Orbit Euler Angs (deg)"
  [ITRF2BodyQ] -> Quaternions to Rotation Angles (Euler)5/1
  [Orbit2BodyDCM] -> TMs Bus Creator/3  "Orbit to Body TM"
  Trigonometric Function1/1 -> Radians to Degrees/1
  Quaternions to Rotation Angles (Euler)4/1 -> Euler Angles Bus Creator/3  "Orbit to Body Euler Angs (deg)"
  [ICRF2BodyDCM] -> Direction Cosine Matrix to Quaternions/1  "ICRF to Body TM"
  [Orbit2BodyDCM] -> ICRF to Body Transfer Matrix Calculator/1

== system SPARCS_MIL/Sensors ==
  Calendar : Inport
  Input1 : Inport  Port=2
  Input3 : Inport  Port=3
  Input4 : Inport  Port=4
  Input6 : Inport  Port=5
  Input7 : Inport  Port=6
  Input8 : Inport  Port=7
  Input9 : Inport  Port=8
  Input10 : Inport  Port=9
  Input11 : Inport  Port=10
  Input12 : Inport  Port=11
  Input13 : Inport  Port=12
  Bus Creator : BusCreator  Inputs=3
  Bus Selector : BusSelector  OutputSignals=signal1,signal2
  GNSS Receiver Model : Subsystem
  Gyroscope Model : Subsystem
  Magnetometer Model : Subsystem
  Sun Sensor Model : Subsystem
  SunPos_Meas(Body) : Outport
  SunPos_Meas(Body)2 : Outport  Port=2
  Power (W) : Outport  Port=3
  wires:
  Calendar/1 -> GNSS Receiver Model/1(Calendar)
  Input1/1 -> GNSS Receiver Model/2(Satellite Ephemeris)
  Input3/1 -> GNSS Receiver Model/4(Sensor Switch)
  Input4/1 -> Gyroscope Model/1(Angular Velocity [Body] (rad/s))
  Input6/1 -> Gyroscope Model/3(Measurement Model DCM)
  Input7/1 -> Gyroscope Model/4(Sensor Switch)
  Input8/1 -> Magnetometer Model/1(Magnetic Field [Body] (T))
  Input9/1 -> Magnetometer Model/2(Temperature (˚C))
  Input10/1 -> Magnetometer Model/3(Input Voltage (V))
  Input11/1 -> Magnetometer Model/4(Measurement Model DCM)
  Input12/1 -> Magnetometer Model/5(Sensor Switch)
  Input13/1 -> Sun Sensor Model/1(Eclipse)
  Sun Sensor Model/1(SunPos_Meas[Body]) -> SunPos_Meas(Body)/1
  Magnetometer Model/2(Power (W)) -> Bus Creator/3  "Magnetometer Power (W)"
  Magnetometer Model/1(Magnetic Field [Sensor](T)) -> SunPos_Meas(Body)2/1
  Gyroscope Model/2(Power (W)) -> Bus Creator/2  "Gyro Power (W)"
  GNSS Receiver Model/2(Power (W)) -> Bus Creator/1  "Power GNSS Receiver (W)"
  Bus Creator/1 -> Power (W)/1
  Bus Selector/1 -> GNSS Receiver Model/3(Input Voltage (V))  "<signal1>"
  Bus Selector/2 -> Gyroscope Model/2(Input Voltage (V))  "<signal2>"
